simulink model "DCmotor"  (R2017a)
settings: Solver=VariableStepAuto  StartTime=0.0  StopTime=2  RelTol=1e-3
values from neighbouring files (symbols this model uses):
  B = 0.1    [Assignment8_case1.m]    (also in Assignment8_case2.m; Assignment8_case3.m; Assignment8_case4.m; Assignment8_case5.m)
  FV = 10    [Assignment8_case1.m]    (also in Assignment8_case2.m = 900; Assignment8_case3.m; Assignment8_case4.m; Assignment8_case5.m)
  J = 0.01    [Assignment8_case1.m]    (also in Assignment8_case2.m; Assignment8_case3.m; Assignment8_case4.m; Assignment8_case5.m)
  K = 0.1    [Assignment8_case1.m]    (also in Assignment8_case2.m; Assignment8_case3.m; Assignment8_case4.m; Assignment8_case5.m)
  La = 0.5e-3    (= 0.0005)    [Assignment8_case1.m]    (also in Assignment8_case2.m; Assignment8_case3.m; Assignment8_case4.m; Assignment8_case5.m)
  Ra = 10    [Assignment8_case1.m]    (also in Assignment8_case2.m; Assignment8_case3.m; Assignment8_case4.m; Assignment8_case5.m)
  Step = 0    [Assignment8_case1.m]    (also in Assignment8_case2.m; Assignment8_case3.m; Assignment8_case4.m; Assignment8_case5.m)
settings Model: Creator=jms2299  LastModifiedBy=jms2299

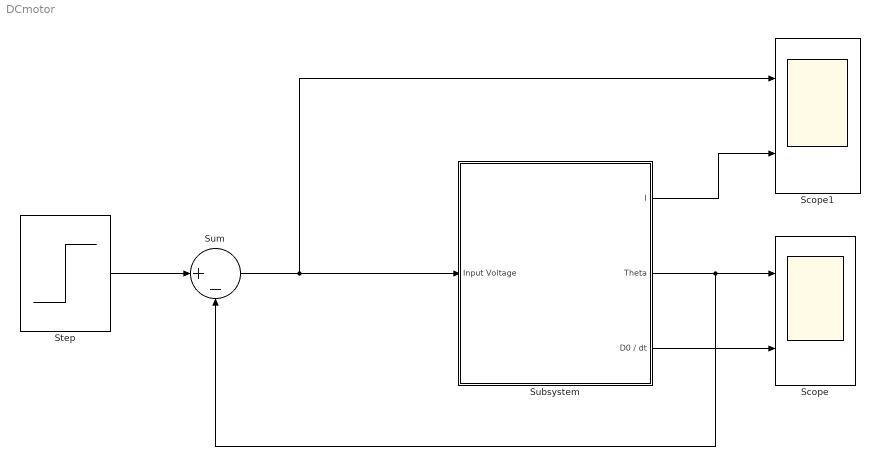
== system DCmotor ==
  Scope : Scope  NumInputPorts=2
  Scope1 : Scope  NumInputPorts=2
  Step : Step  Time=Step  After=FV  SampleTime=0
  Subsystem : Subsystem
  Sum : Sum  Inputs=|+-
  wires:
  Subsystem/1(I) -> Scope1/2
  Subsystem/3(D0 / dt) -> Scope/2
  Subsystem/2(Theta) -> Sum/2, Scope/1
  Step/1 -> Sum/1
  Sum/1 -> Scope1/1, Subsystem/1(Input Voltage)

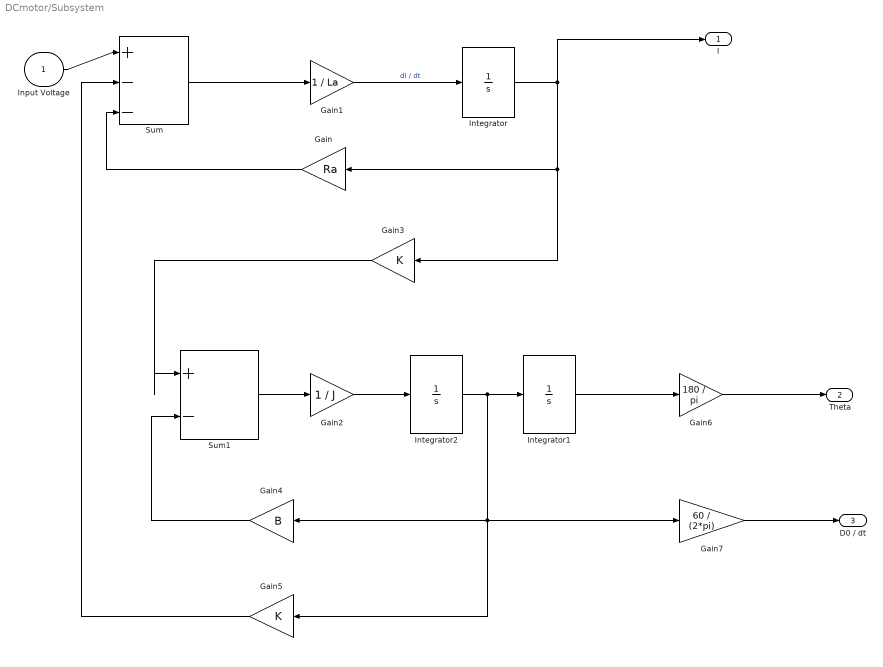
== system DCmotor/Subsystem ==
  Input Voltage : Inport
  Gain : Gain  Gain=Ra
  Gain1 : Gain  Gain=1 / La
  Gain2 : Gain  Gain=1 / J
  Gain3 : Gain  Gain=K
  Gain4 : Gain  Gain=B
  Gain5 : Gain  Gain=K
  Gain6 : Gain  Gain=180 / pi
  Gain7 : Gain  Gain=60 / (2*pi)
  Integrator : Integrator
  Integrator1 : Integrator
  Integrator2 : Integrator
  Sum : Sum  Inputs=|+--
  Sum1 : Sum  Inputs=|+-
  I : Outport
  Theta : Outport  Port=2
  D0 / dt : Outport  Port=3
  wires:
  Sum1/1 -> Gain2/1
  Integrator/1 -> I/1, Gain3/1, Gain/1
  Gain3/1 -> Sum1/1
  Gain/1 -> Sum/3
  Gain1/1 -> Integrator/1  "dI / dt"
  Gain2/1 -> Integrator2/1
  Sum/1 -> Gain1/1
  Gain4/1 -> Sum1/2
  Gain5/1 -> Sum/2
  Integrator2/1 -> Gain7/1, Gain4/1, Gain5/1, Integrator1/1
  Input Voltage/1 -> Sum/1
  Integrator1/1 -> Gain6/1
  Gain6/1 -> Theta/1
  Gain7/1 -> D0 / dt/1
